simulink library "Library_SII_2018"  (R2018b)
settings: Solver=ode45  StartTime=0.0  StopTime=10.0  RelTol=1e-3  EnableMultiTasking=on
undefined symbols (not defined in the file or in its folder): coder, gcbh, r, simscape
libraries: fl_lib x157, nesl_utility x81, Library_SII2 x44, simulink x17, powerlib x12, mblibv1 x11, Simscape_SII_lib x11, elec_lib x10, Pneumatic_lib x4, $bdroot x2, peRmsMeasurement x1, powerlib_extras x1
(part 3 of 6)

== system Library_SII_2018/Electromécanique/Commande moteur Position ==
  cons pos : Inport
  pos codeur : Inport  Port=2
  Abs : Abs
  Constant : Constant  Value=0
  Controlled Voltage Source : fl_lib/Electrical/Electrical Sources/Controlled Voltage Source
  PID Controller : simulink/Continuous/PID Controller  Controller=PID  Form=Parallel  TimeDomain=Continuous-time  SampleTime=-1  IntegratorMethod=Forward Euler  FilterMethod=Forward Euler  ControllerParametersSource=internal  P=P  I=I  D=D  UseFilter=on  N=100  TunerSelectOption=Transfer Function Based (PID Tuner App)  InitialConditionSource=internal  InitialConditionForIntegrator=0  InitialConditionForFilter=0  DifferentiatorICPrevScaledInput=0  ExternalReset=either  TrackingMode=off  Kt=1  LimitOutput=on  UpperSaturationLimit=Umax  LowerSaturationLimit=-Umax  LinearizeAsGain=on  AntiWindupMode=none  Kb=1  POutMin=[]  POutMax=[]  IOutMin=[]  IOutMax=[]  DOutMin=[]  DOutMax=[]  NOutMin=[]  NOutMax=[]  SumOutMin=[]  SumOutMax=[]  SaturationOutMin=[]  SaturationOutMax=[]  PParamMin=[]  PParamMax=[]  IParamMin=[]  IParamMax=[]  DParamMin=[]  DParamMax=[]  NParamMin=[]  NParamMax=[]  KbParamMin=[]  KbParamMax=[]  KtParamMin=[]  KtParamMax=[]  KbOutMin=[]  KbOutMax=[]  KtOutMin=[]  KtOutMax=[]  IntegratorOutMin=[]  IntegratorOutMax=[]  FilterOutMin=[]  FilterOutMax=[]  SumI1OutMin=[]  SumI1OutMax=[]  SumI2OutMin=[]  SumI2OutMax=[]  SumI3OutMin=[]  SumI3OutMax=[]  SumI4OutMin=[]  SumI4OutMax=[]  SumDOutMin=[]  SumDOutMax=[]  DifferentiatorOutMin=[]  DifferentiatorOutMax=[]  FilterDiffOutCoefMin=[]  FilterDiffOutCoefMax=[]  ReciprocalOutMin=[]  ReciprocalOutMax=[]  SumDenOutMin=[]  SumDenOutMax=[]  SumNumOutMin=[]  SumNumOutMax=[]  DivideOutMin=[]  DivideOutMax=[]  IntegratorContinuousStateAttributes=''  IntegratorStateMustResolveToSignalObject=off  IntegratorRTWStateStorageClass=Auto  FilterContinuousStateAttributes=''  FilterStateMustResolveToSignalObject=off  FilterRTWStateStorageClass=Auto  ParallelPVariant=InternalParameters  IdealPVariant=Disabled  IVariant=InternalParameters  DVariant=InternalParameters  IntegratorVariant=Continuous  SatVariant=Enabled  AWVariant=Passthrough  PCopyVariant=Disabled  TRVariant=Disabled  FdbkBlocksVariant=Forward  IdealPFdbkVariant=Disabled  SatFdbkVariant=Disabled  DerivativeFilterVariant=ContFilter  NVariant=InternalParameters  NCopyVariant=Disabled  FilterICVariant=InternalICsFilter  IntegratorICVariant=InternalICs  ExternalResetVariant=ExternalReset  TRSumVariant=Passthrough  SumFdbkVariant=Disabled  SumVariant=Sum_PID
  Relay : Relay  OnSwitchValue=e  OffSwitchValue=e/2
  Simulink-PS Converter1 : nesl_utility/Simulink-PS Converter  PhysicalDomain=network_engine_domain  SubClassName=ps_input  LeftPortType=input  RightPortType=output  PseudoPeriodic=off  Frequencies=[]  NoiseDistribution=none  NoiseParameters=[]  Unit=1  AffineConversion=off  FilteringAndDerivatives=zero  SimscapeFilterOrder=1  InputFilterTimeConstant=0.001  UdotUserProvided=1
  Sum : Sum  Inputs=|+-
  Switch : Switch  Criteria=u2 > Threshold
  +mot : PMIOPort  Side=Right
  GND : PMIOPort  Port=2  Side=Right
  wires:
  pos codeur/1 -> Sum/2
  Switch/1 -> Simulink-PS Converter1/1, PID Controller/2
  Sum/1 -> Abs/1, PID Controller/1
  cons pos/1 -> Sum/1
  Constant/1 -> Switch/3
  Abs/1 -> Relay/1
  PID Controller/1 -> Switch/1
  Relay/1 -> Switch/2
  connections:
  GND/RConn1 -- Controlled Voltage Source/RConn2
  +mot/RConn1 -- Controlled Voltage Source/LConn1
  Simulink-PS Converter1/RConn1 -- Controlled Voltage Source/RConn1

== system Library_SII_2018/Electromécanique/Décodeur pour codeur incrémental ==
  A : Inport
  B : Inport  Port=2
  Clock1 : Clock
  Décodeur position - vitesse accélération - fréquence : Stateflow chart  TreatAsAtomicUnit=on
  MATLAB Function : MATLAB Function  TreatAsAtomicUnit=on
  Résolution : Constant  Value=r/2
  Terminator : Terminator
  Terminator1 : Terminator
  Terminator2 : Terminator
  inversion : Constant  Value=inv
  pos codeur : Outport
  wires:
  A/1 -> Décodeur position - vitesse accélération - fréquence/1(A), Décodeur position - vitesse accélération - fréquence/Trigger
  Clock1/1 -> Décodeur position - vitesse accélération - fréquence/4(t)
  B/1 -> Décodeur position - vitesse accélération - fréquence/2(B)
  Résolution/1 -> MATLAB Function/1(u)
  Décodeur position - vitesse accélération - fréquence/1(p) -> pos codeur/1
  Décodeur position - vitesse accélération - fréquence/2(v) -> Terminator/1
  Décodeur position - vitesse accélération - fréquence/4(f) -> Terminator2/1
  Décodeur position - vitesse accélération - fréquence/3(a) -> Terminator1/1
  MATLAB Function/1(y) -> Décodeur position - vitesse accélération - fréquence/3(k)
  inversion/1 -> MATLAB Function/2(inv)

== system Library_SII_2018/Electromécanique/Moteur CC (SPS-SM) ==
  Actionneur en vitesse : Subsystem
  Axe (inertie nulle) : mblibv1/Bodies/Body  LConnTagsString=CG  RConnTagsString=CS2  UpdateFromCAD=off  DialogClass=MechanicalBodyBlock  Mass=0.0001  MassUnits=kg  InertiaUnits=kg*m^2  Inertia=[1e-9 0 0 ; 0 1e-8 0 ; 0 0 1e-8]  Shape=Cylinder  ShapeDims=[1 1]  ShapeUnits=m  ShapeUse=false  Density=1  DensityUnits=kg/m^3  DensityUse=false  GraphicsMode=EQELLIPSE  BodyColorSelMode=COLORPALETTE  BodyColor=[0 1 0]  AttachedToCS=CG  CG=Left$CG$[0 0 0]$Adjoining$Adjoining$m$[0 0 0]$Euler X-Y-Z$deg$World$true$none  WorkingFrames=Right$CS2$[0 0 0]$CG$CG$mm$[0 0 0]$Euler X-Y-Z$deg$World$true$none  CGPos=[0 0 0]  CGRot=[0 0 0]  CS0Pos=[]  CS0Rot=[]  CS1Pos=[]  CS1Rot=[]  CS2Pos=[0 0 0]  CS2Rot=[0 0 0]  CS3Pos=[]  CS3Rot=[]  CS4Pos=[]  CS4Rot=[]  CS5Pos=[]  CS5Rot=[]  CS6Pos=[]  CS6Rot=[]  CS7Pos=[]  CS7Rot=[]  CS8Pos=[]  CS8Rot=[]  CS9Pos=[]  CS9Rot=[]  CS10Pos=[]  CS10Rot=[]  CS11Pos=[]  CS11Rot=[]  CS12Pos=[]  CS12Rot=[]  CS13Pos=[]  CS13Rot=[]  CS14Pos=[]  CS14Rot=[]  CS15Pos=[]  CS15Rot=[]  CS16Pos=[]  CS16Rot=[]  CS17Pos=[]  CS17Rot=[]  CS18Pos=[]  CS18Rot=[]  CS19Pos=[]  CS19Rot=[]  CS20Pos=[]  CS20Rot=[]
      settings: SourceProductName=Simscape Multibody  SourceProductBaseCode=MS
  Bus Selector : BusSelector  OutputSignals=Electrical torque Te (n m),Speed wm (rad/s)
  Capteur de couple : mblibv1/Sensors &  Actuators/Joint Sensor  UpdateFromCAD=off  PhysicalDomain=Mechanical  PortType=blob  Muxed=on  Pose=off  Angle=off  AngleUnits=deg  ArcVelocity=off  ArcVelocityUnits=deg/s  ArcAcceleration=off  ArcAccelerationUnits=deg/s^2  CoordPosition=on  CoordPositionUnits=m  Velocity=off  VelocityUnits=m/s  Acceleration=off  AccelerationUnits=m/s^2  Quaternion=on  QuaternionDT=off  QuaternionDDT=off  QuaternionUnits=off  OutputVector=[1]  ActiveIO=off  Width=3  DialogClass=MechanicalSensorBlock  Primitive=W  Force=off  ForceUnits=N  Torque=on  TorqueUnits=N*m  ReferenceFrame=Absolute (World)  ReactionSensedSide=Base  ReactionReferenceFrame=Absolute (World)  ReactionForce=off  ReactionForceUnits=N  ReactionMoment=on  ReactionMomentUnits=N*m
      settings: SourceProductName=Simscape Multibody  SourceProductBaseCode=MS
  Couple résistant : Scope
  Couple moteur : Scope
  DC Machine : powerlib/Machines/DC Machine  PresetModel=No  MechanicalLoad=Torque TL  FieldType=Permanent magnet  ShowDetailedParameters=on  MeasurementBus=off  RLa=[R L]  RLf=[281.3 156]  Laf=0.9483  MachineConstant=Back-emf constant (V/rpm)  Ke=K  Kt=1.8  J=J  Bm=kv  Tf=kc  w0=0  Ifinit=1  TsPowergui=0  TsBlock=-1
      settings: AttributesFormatString=\n  SourceProductName=Simscape Electrical
  Demux : Demux  Outputs=3
  Encastrement : mblibv1/Joints/Weld  LConnTagsString=__newl0|SA1  RConnTagsString=__newr0  UpdateFromCAD=off  NumSAPorts=1  CutJoint=off  MarkAsCut=off  Primitives=weld  PrimitiveProps=W$World$[0 0 0]$weld  DialogClass=JointBlock  WAxis=[0 0 0]
      settings: SourceProductName=Simscape Multibody  SourceProductBaseCode=MS
  Gain : Gain  Gain=-1
  Revolute : mblibv1/Joints/Revolute  LConnTagsString=__newl0|SA1  RConnTagsString=__newr0  UpdateFromCAD=off  NumSAPorts=1  CutJoint=off  MarkAsCut=off  Primitives=prismatic  PrimitiveProps=R1$World$[1 0 0]$revolute  DialogClass=JointBlock  R1Axis=[1 0 0]
      settings: SourceProductName=Simscape Multibody  SourceProductBaseCode=MS
  T : Terminator
  T1 : Terminator
  Stator : PMIOPort  Side=Left
  Rotor : PMIOPort  Port=2  Side=Right
  A+ : PMIOPort  Port=3  Side=Left
  A- : PMIOPort  Port=4  Side=Right
  wires:
  Bus Selector/2 -> Actionneur en vitesse/1(signal)  "<Speed wm (rad/s)>"
  Demux/3 -> T1/1
  Demux/2 -> T/1  "Couple"
  Demux/1 -> Gain/1
  Gain/1 -> Couple résistant/1, DC Machine/1
  Bus Selector/1 -> Couple moteur/1  "<Electrical torque Te (n m)>"
  Capteur de couple/1 -> Demux/1
  DC Machine/1 -> Bus Selector/1
  connections:
  A-/RConn1 -- DC Machine/RConn1
  A+/RConn1 -- DC Machine/LConn1
  Stator/RConn1 -- Revolute/LConn1
  Actionneur en vitesse/RConn1 -- Revolute/LConn2
  Encastrement/RConn1 -- Rotor/RConn1
  Capteur de couple/LConn1 -- Encastrement/LConn2
  Axe (inertie nulle)/RConn1 -- Encastrement/LConn1
  Revolute/RConn1 -- Axe (inertie nulle)/LConn1

== system Library_SII_2018/Electromécanique/Moteur CC (SPS-SS) ==
  Bus Selector : BusSelector  OutputSignals=Electrical torque Te (n m),Speed wm (rad/s)
  Capteur de couple : fl_lib/Mechanical/Mechanical Sensors/Ideal Torque Sensor
  Couple résistant : Scope
  Couple moteur : Scope
  DC Machine : powerlib/Machines/DC Machine  PresetModel=No  MechanicalLoad=Torque TL  FieldType=Permanent magnet  ShowDetailedParameters=on  MeasurementBus=off  RLa=[R L]  RLf=[281.3 156]  Laf=0.9483  MachineConstant=Back-emf constant (V/rpm)  Ke=K  Kt=1.8  J=J  Bm=kv  Tf=kc  w0=0  Ifinit=1  TsPowergui=0  TsBlock=-1
      settings: AttributesFormatString=\n  SourceProductName=Simscape Electrical
  Frottement visqueux : fl_lib/Mechanical/Rotational Elements/Rotational Damper  D=kv N*m/(rad/s)  w_specify=off  w_priority=High  w=0 rad/s  w_nominal_specify=off  w_nominal_unit=rad/s  w_nominal_value=1  t_specify=off  t_priority=High  t=0 N*m  t_nominal_specify=off  t_nominal_unit=N*m  t_nominal_value=1
  Gain : Gain  Gain=-1
  Inertie arbre : fl_lib/Mechanical/Rotational Elements/Inertia  inertia=J kg*m^2  w_specify=on  w_priority=High  w=0 rad/s  w_nominal_specify=off  w_nominal_unit=rad/s  w_nominal_value=1  t_specify=off  t_priority=High  t=0 N*m  t_nominal_specify=off  t_nominal_unit=N*m  t_nominal_value=1
  Mechanical Rotational Reference : fl_lib/Mechanical/Rotational Elements/Mechanical Rotational Reference
  PS-Simulink Converter : nesl_utility/PS-Simulink Converter  PhysicalDomain=network_engine_domain  SubClassName=ps_output  LeftPortType=input  RightPortType=output  PseudoPeriodic=off  Frequencies=[]  Unit=1  AffineConversion=off
  Ref : fl_lib/Mechanical/Rotational Elements/Mechanical Rotational Reference
  Ref Stator : fl_lib/Mechanical/Rotational Elements/Mechanical Rotational Reference
  Simulink-PS Converter : nesl_utility/Simulink-PS Converter  PhysicalDomain=network_engine_domain  SubClassName=ps_input  LeftPortType=input  RightPortType=output  PseudoPeriodic=off  Frequencies=[]  NoiseDistribution=none  NoiseParameters=[]  Unit=1  AffineConversion=off  FilteringAndDerivatives=zero  SimscapeFilterOrder=1  InputFilterTimeConstant=.001  UdotUserProvided=0
  Solver Configuration : nesl_utility/Solver Configuration  PhysicalDomain=network_engine_domain  SubClassName=solver  LeftPortType=input  RightPortType=generic  Tones=[]  Harmonics=[]  SimulateNoise=off  Profile=off  UseLocalSampling=off  EnableSwitchedLinearOptims=on  FrequencyDomain=off  UseCCode=off  RelTol=0.001  AbsTol=1e-06  MinStep=1e-09  ToWorkspace=off  RevertToSquareIcSolve=off  NumHomotopyIterations=100  PhasorMode=off  PhasorModeNumHarmonics=1  DoDC=off  ResidualTolerance=1e-9  UseLocalSolver=off  LocalSolverChoice=NE_BACKWARD_EULER_ADVANCER  LocalSolverSampleTime=.001  DoFixedCost=off  MaxNonlinIter=3  MaxModeIter=2  LinearAlgebra=Sparse  EquationFormulation=NE_TIME_EF  DelaysMemoryBudget=1024  AutomaticFiltering=on  FilteringTimeConstant=0.001  PartitionStorageMethod=AS_NEEDED  PartitionMemoryBudget=1024
  Source de vitesse : fl_lib/Mechanical/Mechanical Sources/Ideal Angular Velocity Source
  Stator : PMIOPort  Side=Left
  Rotor : PMIOPort  Port=2  Side=Right
  A+ : PMIOPort  Port=3  Side=Left
  A- : PMIOPort  Port=4  Side=Right
  wires:
  Bus Selector/2 -> Simulink-PS Converter/1  "<Speed wm (rad/s)>"
  PS-Simulink Converter/1 -> Gain/1
  Gain/1 -> Couple résistant/1, DC Machine/1
  Bus Selector/1 -> Couple moteur/1  "<Electrical torque Te (n m)>"
  DC Machine/1 -> Bus Selector/1
  connections:
  Capteur de couple/RConn1 -- Source de vitesse/LConn1 -- Frottement visqueux/RConn1 -- Inertie arbre/LConn1
  Mechanical Rotational Reference/LConn1 -- Source de vitesse/RConn2
  Ref/LConn1 -- Frottement visqueux/LConn1
  Capteur de couple/LConn1 -- Solver Configuration/RConn1 -- Rotor/RConn1
  Capteur de couple/RConn2 -- PS-Simulink Converter/LConn1
  Ref Stator/LConn1 -- Stator/RConn1
  Source de vitesse/RConn1 -- Simulink-PS Converter/RConn1
  A-/RConn1 -- DC Machine/RConn1
  A+/RConn1 -- DC Machine/LConn1

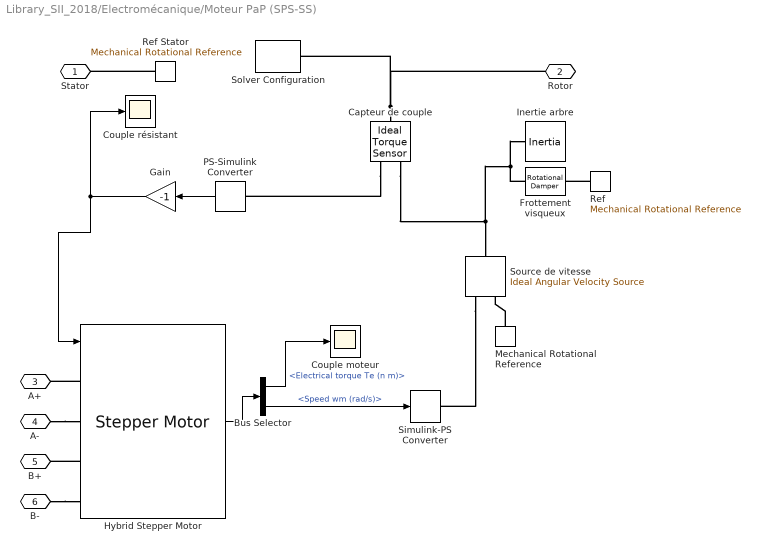
== system Library_SII_2018/Electromécanique/Moteur PaP (SPS-SS) ==
  Bus Selector : BusSelector  OutputSignals=Electrical torque Te (n m),Speed wm (rad/s)
  Capteur de couple : fl_lib/Mechanical/Mechanical Sensors/Ideal Torque Sensor
  Couple résistant : Scope
  Couple moteur : Scope
  Frottement visqueux : fl_lib/Mechanical/Rotational Elements/Rotational Damper  D=kv N*m/(rad/s)  w_specify=off  w_priority=High  w=0 rad/s  w_nominal_specify=off  w_nominal_unit=rad/s  w_nominal_value=1  t_specify=off  t_priority=High  t=0 N*m  t_nominal_specify=off  t_nominal_unit=N*m  t_nominal_value=1
  Gain : Gain  Gain=-1
  Hybrid Stepper Motor : powerlib/Machines/Stepper Motor  MotorType=Permanent-magnet / Hybrid  NumberOfPhases_1=2  NumberOfPhases_2=3  PresetModel_1=<empty>  PresetModel_2=<empty>  L=1.4e-3  Lmax=10e-3  Lmin=2e-3  R=0.7  Step_angle=1.8  Psim=0.005  Tdm=0.002  J=1.2e-7  B=1e-7*1000  w0=0  pos0=0  TsPowergui=0  TsBlock=-1
      settings: SourceProductName=Simscape Electrical  SourceProductBaseCode=PS
  Inertie arbre : fl_lib/Mechanical/Rotational Elements/Inertia  inertia=J kg*m^2  w_specify=on  w_priority=High  w=0 rad/s  w_nominal_specify=off  w_nominal_unit=rad/s  w_nominal_value=1  t_specify=off  t_priority=High  t=0 N*m  t_nominal_specify=off  t_nominal_unit=N*m  t_nominal_value=1
  Mechanical Rotational Reference : fl_lib/Mechanical/Rotational Elements/Mechanical Rotational Reference
  PS-Simulink Converter : nesl_utility/PS-Simulink Converter  PhysicalDomain=network_engine_domain  SubClassName=ps_output  LeftPortType=input  RightPortType=output  PseudoPeriodic=off  Frequencies=[]  Unit=1  AffineConversion=off
  Ref : fl_lib/Mechanical/Rotational Elements/Mechanical Rotational Reference
  Ref Stator : fl_lib/Mechanical/Rotational Elements/Mechanical Rotational Reference
  Simulink-PS Converter : nesl_utility/Simulink-PS Converter  PhysicalDomain=network_engine_domain  SubClassName=ps_input  LeftPortType=input  RightPortType=output  PseudoPeriodic=off  Frequencies=[]  NoiseDistribution=none  NoiseParameters=[]  Unit=1  AffineConversion=off  FilteringAndDerivatives=zero  SimscapeFilterOrder=1  InputFilterTimeConstant=.001  UdotUserProvided=0
  Solver Configuration : nesl_utility/Solver Configuration  PhysicalDomain=network_engine_domain  SubClassName=solver  LeftPortType=input  RightPortType=generic  Tones=[]  Harmonics=[]  SimulateNoise=off  Profile=off  UseLocalSampling=off  EnableSwitchedLinearOptims=on  FrequencyDomain=off  UseCCode=off  RelTol=0.001  AbsTol=1e-06  MinStep=1e-09  ToWorkspace=off  RevertToSquareIcSolve=off  NumHomotopyIterations=100  PhasorMode=off  PhasorModeNumHarmonics=1  DoDC=off  ResidualTolerance=1e-9  UseLocalSolver=off  LocalSolverChoice=NE_BACKWARD_EULER_ADVANCER  LocalSolverSampleTime=.001  DoFixedCost=off  MaxNonlinIter=3  MaxModeIter=2  LinearAlgebra=Sparse  EquationFormulation=NE_TIME_EF  DelaysMemoryBudget=1024  AutomaticFiltering=on  FilteringTimeConstant=0.001  PartitionStorageMethod=AS_NEEDED  PartitionMemoryBudget=1024
  Source de vitesse : fl_lib/Mechanical/Mechanical Sources/Ideal Angular Velocity Source
  Stator : PMIOPort  Side=Left
  Rotor : PMIOPort  Port=2  Side=Right
  A+ : PMIOPort  Port=3  Side=Left
  A- : PMIOPort  Port=4  Side=Right
  B+ : PMIOPort  Port=5  Side=Left
  B- : PMIOPort  Port=6  Side=Right
  wires:
  Bus Selector/2 -> Simulink-PS Converter/1  "<Speed wm (rad/s)>"
  PS-Simulink Converter/1 -> Gain/1
  Gain/1 -> Hybrid Stepper Motor/1, Couple résistant/1
  Bus Selector/1 -> Couple moteur/1  "<Electrical torque Te (n m)>"
  Hybrid Stepper Motor/1 -> Bus Selector/1
  connections:
  Capteur de couple/RConn1 -- Source de vitesse/LConn1 -- Frottement visqueux/RConn1 -- Inertie arbre/LConn1
  Mechanical Rotational Reference/LConn1 -- Source de vitesse/RConn2
  Ref/LConn1 -- Frottement visqueux/LConn1
  Capteur de couple/LConn1 -- Solver Configuration/RConn1 -- Rotor/RConn1
  Capteur de couple/RConn2 -- PS-Simulink Converter/LConn1
  Ref Stator/LConn1 -- Stator/RConn1
  Source de vitesse/RConn1 -- Simulink-PS Converter/RConn1
  A-/RConn1 -- Hybrid Stepper Motor/LConn2
  Hybrid Stepper Motor/LConn1 -- A+/RConn1
  Hybrid Stepper Motor/LConn3 -- B+/RConn1
  B-/RConn1 -- Hybrid Stepper Motor/LConn4

== system Library_SII_2018/Electromécanique/Pont en H ==
  mode : Inport
  Commande du pont en H : MATLAB Function  TreatAsAtomicUnit=on
  Simulink-PS Converter{1,3..5} (4 alike) : nesl_utility/Simulink-PS Converter  PhysicalDomain=network_engine_domain  SubClassName=ps_input  LeftPortType=input  RightPortType=output  PseudoPeriodic=off  Frequencies=[]  NoiseDistribution=none  NoiseParameters=[]  Unit=V  AffineConversion=off  FilteringAndDerivatives=zero  SimscapeFilterOrder=1  InputFilterTimeConstant=0.1  UdotUserProvided=1
  a : fl_lib/Electrical/Electrical Elements/Switch  R_closed=0.01 Ohm  G_open=1e-8 1/Ohm  Threshold=0.5  i_specify=off  i_priority=High  i=0 A  i_nominal_specify=off  i_nominal_unit=A  i_nominal_value=1  v_specify=off  v_priority=High  v=0 V  v_nominal_specify=off  v_nominal_unit=V  v_nominal_value=1
      settings: SourceProductName=Simscape
  b : fl_lib/Electrical/Electrical Elements/Switch  R_closed=0.01 Ohm  G_open=1e-8 1/Ohm  Threshold=0.5  i_specify=off  i_priority=High  i=0 A  i_nominal_specify=off  i_nominal_unit=A  i_nominal_value=1  v_specify=off  v_priority=High  v=0 V  v_nominal_specify=off  v_nominal_unit=V  v_nominal_value=1
      settings: SourceProductName=Simscape
  c : fl_lib/Electrical/Electrical Elements/Switch  R_closed=0.01 Ohm  G_open=1e-8 1/Ohm  Threshold=0.5  i_specify=off  i_priority=High  i=0 A  i_nominal_specify=off  i_nominal_unit=A  i_nominal_value=1  v_specify=off  v_priority=High  v=0 V  v_nominal_specify=off  v_nominal_unit=V  v_nominal_value=1
      settings: SourceProductName=Simscape
  d : fl_lib/Electrical/Electrical Elements/Switch  R_closed=0.01 Ohm  G_open=1e-8 1/Ohm  Threshold=0.5  i_specify=off  i_priority=High  i=0 A  i_nominal_specify=off  i_nominal_unit=A  i_nominal_value=1  v_specify=off  v_priority=High  v=0 V  v_nominal_specify=off  v_nominal_unit=V  v_nominal_value=1
      settings: SourceProductName=Simscape
  Vcc : PMIOPort  Side=Left
  +Mot : PMIOPort  Port=2  Side=Right
  -Mot : PMIOPort  Port=3  Side=Right
  Ref : PMIOPort  Port=4  Side=Left
  wires:
  Commande du pont en H/1(a) -> Simulink-PS Converter1/1
  Commande du pont en H/3(c) -> Simulink-PS Converter5/1
  Commande du pont en H/4(d) -> Simulink-PS Converter4/1
  mode/1 -> Commande du pont en H/1(mode)
  Commande du pont en H/2(b) -> Simulink-PS Converter3/1
  connections:
  a/LConn1 -- +Mot/RConn1 -- c/RConn2
  Simulink-PS Converter1/RConn1 -- a/RConn1
  Simulink-PS Converter5/RConn1 -- c/RConn1
  b/RConn2 -- Vcc/RConn1 -- a/RConn2
  Simulink-PS Converter3/RConn1 -- b/RConn1
  d/LConn1 -- Ref/RConn1 -- c/LConn1
  Simulink-PS Converter4/RConn1 -- d/RConn1
  b/LConn1 -- -Mot/RConn1 -- d/RConn2

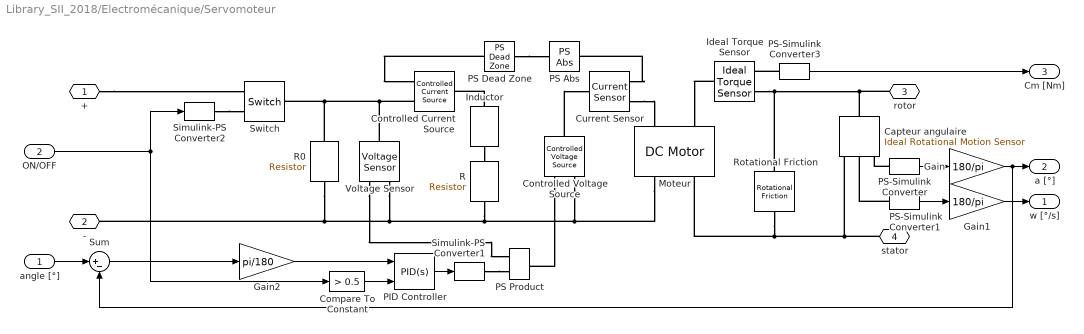
== system Library_SII_2018/Electromécanique/Servomoteur ==
  angle [°] : Inport
  ON/OFF : Inport  Port=2
  Capteur angulaire : fl_lib/Mechanical/Mechanical Sensors/Ideal Rotational Motion Sensor  offset=0 rad
  Compare To Constant : simulink/Logic and Bit Operations/Compare To Constant  relop=>  const=0.5  OutDataTypeStr=boolean
  Controlled Current Source : fl_lib/Electrical/Electrical Sources/Controlled Current Source
  Controlled Voltage Source : fl_lib/Electrical/Electrical Sources/Controlled Voltage Source
  Current Sensor : fl_lib/Electrical/Electrical Sensors/Current Sensor
  Gain : Gain  Gain=180/pi
  Gain1 : Gain  Gain=180/pi
  Gain2 : Gain  Gain=pi/180
  Ideal Torque Sensor : fl_lib/Mechanical/Mechanical Sensors/Ideal Torque Sensor
  Inductor : fl_lib/Electrical/Electrical Elements/Inductor  l=L H  r=0 Ohm  g=1e-9 1/Ohm  i_specify=off  i_priority=High  i=0 A  i_nominal_specify=off  i_nominal_unit=A  i_nominal_value=1  v_specify=off  v_priority=High  v=0 V  v_nominal_specify=off  v_nominal_unit=V  v_nominal_value=1  i_L_specify=off  i_L_priority=High  i_L=0 A  i_L_nominal_specify=off  i_L_nominal_unit=A  i_L_nominal_value=1
  Moteur : elec_lib/Actuators & Drivers/Rotational Actuators/DC Motor  parameterization=1  Ra=R Ohm  La=L H  emf_or_torque=1  Kv=K V/(rad/s)  Ki=6.876e-4 N*m/A  T_stall=2.4e-4 N*m  w_max=1.91e+4 rpm  w_rated=1.5e+4 rpm  P_rated=0.08 W  V_rated=1.5 V  J=0.001 g*cm^2  lam_param=1  lam=kv N*m/(rad/s)  i_noload=0 A  V_i_noload=1.5 V  speed0=0 rpm  alpha=0.00393 1/K  Tmeas=25 C  thermal_mass=100 J/K  initial_temperature=25 C
  PID Controller : simulink/Continuous/PID Controller  Controller=PID  Form=Ideal  TimeDomain=Continuous-time  SampleTime=-1  IntegratorMethod=Forward Euler  FilterMethod=Forward Euler  ControllerParametersSource=internal  P=P  I=I  D=D  UseFilter=on  N=100  TunerSelectOption=Transfer Function Based (PID Tuner App)  InitialConditionSource=internal  InitialConditionForIntegrator=0  InitialConditionForFilter=0  DifferentiatorICPrevScaledInput=0  ExternalReset=rising  TrackingMode=off  Kt=1  LimitOutput=on  UpperSaturationLimit=1  LowerSaturationLimit=-1  LinearizeAsGain=on  AntiWindupMode=none  Kb=1  POutMin=[]  POutMax=[]  IOutMin=[]  IOutMax=[]  DOutMin=[]  DOutMax=[]  NOutMin=[]  NOutMax=[]  SumOutMin=[]  SumOutMax=[]  SaturationOutMin=[]  SaturationOutMax=[]  PParamMin=[]  PParamMax=[]  IParamMin=[]  IParamMax=[]  DParamMin=[]  DParamMax=[]  NParamMin=[]  NParamMax=[]  KbParamMin=[]  KbParamMax=[]  KtParamMin=[]  KtParamMax=[]  KbOutMin=[]  KbOutMax=[]  KtOutMin=[]  KtOutMax=[]  IntegratorOutMin=[]  IntegratorOutMax=[]  FilterOutMin=[]  FilterOutMax=[]  SumI1OutMin=[]  SumI1OutMax=[]  SumI2OutMin=[]  SumI2OutMax=[]  SumI3OutMin=[]  SumI3OutMax=[]  SumI4OutMin=[]  SumI4OutMax=[]  SumDOutMin=[]  SumDOutMax=[]  DifferentiatorOutMin=[]  DifferentiatorOutMax=[]  FilterDiffOutCoefMin=[]  FilterDiffOutCoefMax=[]  ReciprocalOutMin=[]  ReciprocalOutMax=[]  SumDenOutMin=[]  SumDenOutMax=[]  SumNumOutMin=[]  SumNumOutMax=[]  DivideOutMin=[]  DivideOutMax=[]  IntegratorContinuousStateAttributes=''  IntegratorStateMustResolveToSignalObject=off  IntegratorRTWStateStorageClass=Auto  FilterContinuousStateAttributes=''  FilterStateMustResolveToSignalObject=off  FilterRTWStateStorageClass=Auto  ParallelPVariant=Passthrough  IdealPVariant=InternalParameters  IVariant=InternalParameters  DVariant=InternalParameters  IntegratorVariant=Continuous  SatVariant=Enabled  AWVariant=Passthrough  PCopyVariant=Disabled  TRVariant=Disabled  FdbkBlocksVariant=Forward  IdealPFdbkVariant=Disabled  SatFdbkVariant=Disabled  DerivativeFilterVariant=ContFilter  NVariant=InternalParameters  NCopyVariant=Disabled  FilterICVariant=InternalICsFilter  IntegratorICVariant=InternalICs  ExternalResetVariant=ExternalReset  TRSumVariant=Passthrough  SumFdbkVariant=Disabled  SumVariant=Sum_PID
  PS Abs : fl_lib/Physical Signals/Nonlinear Operators/PS Abs
      settings: SourceProductName=Simscape  SourceProductBaseCode=SS
  PS Dead Zone : fl_lib/Physical Signals/Nonlinear Operators/PS Dead Zone  upper_limit=0.01  lower_limit=- 0.01
      settings: SourceProductName=Simscape  SourceProductBaseCode=SS
  PS Product : fl_lib/Physical Signals/Functions/PS Product
      settings: SourceProductName=Simscape
  PS-Simulink Converter : nesl_utility/PS-Simulink Converter  PhysicalDomain=network_engine_domain  SubClassName=ps_output  LeftPortType=input  RightPortType=output  PseudoPeriodic=off  Frequencies=[]  Unit=1  AffineConversion=off
  PS-Simulink Converter1 : nesl_utility/PS-Simulink Converter  PhysicalDomain=network_engine_domain  SubClassName=ps_output  LeftPortType=input  RightPortType=output  PseudoPeriodic=off  Frequencies=[]  Unit=1  AffineConversion=off
  PS-Simulink Converter3 : nesl_utility/PS-Simulink Converter  PhysicalDomain=network_engine_domain  SubClassName=ps_output  LeftPortType=input  RightPortType=output  PseudoPeriodic=off  Frequencies=[]  Unit=1  AffineConversion=off
  R : fl_lib/Electrical/Electrical Elements/Resistor  R=R Ohm  i_specify=off  i_priority=High  i=0 A  i_nominal_specify=off  i_nominal_unit=A  i_nominal_value=1  v_specify=off  v_priority=High  v=0 V  v_nominal_specify=off  v_nominal_unit=V  v_nominal_value=1
  R0 : fl_lib/Electrical/Electrical Elements/Resistor  R=R0 Ohm  i_specify=off  i_priority=High  i=0 A  i_nominal_specify=off  i_nominal_unit=A  i_nominal_value=1  v_specify=off  v_priority=High  v=0 V  v_nominal_specify=off  v_nominal_unit=V  v_nominal_value=1
  Rotational Friction : fl_lib/Mechanical/Rotational Elements/Rotational Friction  brkwy_trq=Cf*1.1 N*m  brkwy_vel=0.060623 rad/s  Col_trq=Cf N*m  visc_coef=0.0001 N*m/(rad/s)  w_specify=off  w_priority=High  w=0 rad/s  w_nominal_specify=off  w_nominal_unit=rad/s  w_nominal_value=1  t_specify=off  t_priority=High  t=0 N*m  t_nominal_specify=off  t_nominal_unit=N*m  t_nominal_value=1
      settings: SourceProductName=Simscape
  Simulink-PS Converter1 : nesl_utility/Simulink-PS Converter  PhysicalDomain=network_engine_domain  SubClassName=ps_input  LeftPortType=input  RightPortType=output  PseudoPeriodic=off  Frequencies=[]  NoiseDistribution=none  NoiseParameters=[]  Unit=V  AffineConversion=off  FilteringAndDerivatives=zero  SimscapeFilterOrder=1  InputFilterTimeConstant=0.1  UdotUserProvided=1
  Simulink-PS Converter2 : nesl_utility/Simulink-PS Converter  PhysicalDomain=network_engine_domain  SubClassName=ps_input  LeftPortType=input  RightPortType=output  PseudoPeriodic=off  Frequencies=[]  NoiseDistribution=none  NoiseParameters=[]  Unit=V  AffineConversion=off  FilteringAndDerivatives=zero  SimscapeFilterOrder=1  InputFilterTimeConstant=0.1  UdotUserProvided=1
  Sum : Sum  Inputs=|+-
  Switch : fl_lib/Electrical/Electrical Elements/Switch  R_closed=0.01 Ohm  G_open=1e-8 1/Ohm  Threshold=0.5  i_specify=off  i_priority=High  i=0 A  i_nominal_specify=off  i_nominal_unit=A  i_nominal_value=1  v_specify=off  v_priority=High  v=0 V  v_nominal_specify=off  v_nominal_unit=V  v_nominal_value=1
      settings: SourceProductName=Simscape
  Voltage Sensor : fl_lib/Electrical/Electrical Sensors/Voltage Sensor
  + : PMIOPort  Side=Left
  - : PMIOPort  Port=2  Side=Left
  rotor : PMIOPort  Port=3  Side=Right
  stator : PMIOPort  Port=4  Side=Right
  w [°/s] : Outport
  a [°] : Outport  Port=2
  Cm [Nm] : Outport  Port=3
  wires:
  PID Controller/1 -> Simulink-PS Converter1/1
  Gain1/1 -> w [°/s]/1
  PS-Simulink Converter/1 -> Gain/1
  PS-Simulink Converter1/1 -> Gain1/1
  Gain2/1 -> PID Controller/1
  angle [°]/1 -> Sum/1
  Gain/1 -> Sum/2, a [°]/1
  Sum/1 -> Gain2/1
  ON/OFF/1 -> Simulink-PS Converter2/1, Compare To Constant/1
  Compare To Constant/1 -> PID Controller/2
  PS-Simulink Converter3/1 -> Cm [Nm]/1
  connections:
  Inductor/RConn1 -- R/LConn1
  Inductor/LConn1 -- Controlled Current Source/LConn1
  Current Sensor/RConn1 -- PS Abs/LConn1
  Current Sensor/RConn2 -- Moteur/LConn1
  Controlled Current Source/RConn2 -- Voltage Sensor/LConn1 -- Switch/LConn1 -- R0/LConn1
  Controlled Voltage Source/LConn1 -- Current Sensor/LConn1
  Voltage Sensor/RConn2 -- R/RConn1 -- Controlled Voltage Source/RConn2 -- Moteur/RConn1 -- -/RConn1 -- R0/RConn1
  rotor/RConn1 -- Rotational Friction/LConn1 -- Ideal Torque Sensor/RConn1 -- Capteur angulaire/LConn1
  PS-Simulink Converter/LConn1 -- Capteur angulaire/RConn3
  PS-Simulink Converter1/LConn1 -- Capteur angulaire/RConn2
  Capteur angulaire/RConn1 -- Moteur/RConn2 -- Rotational Friction/RConn1 -- stator/RConn1
  PS Dead Zone/LConn1 -- PS Abs/RConn1
  Controlled Voltage Source/RConn1 -- PS Product/RConn1
  Simulink-PS Converter1/RConn1 -- PS Product/LConn2
  Voltage Sensor/RConn1 -- PS Product/LConn1
  +/RConn1 -- Switch/RConn2
  Simulink-PS Converter2/RConn1 -- Switch/RConn1
  PS Dead Zone/RConn1 -- Controlled Current Source/RConn1
  Ideal Torque Sensor/LConn1 -- Moteur/LConn2
  PS-Simulink Converter3/LConn1 -- Ideal Torque Sensor/RConn2

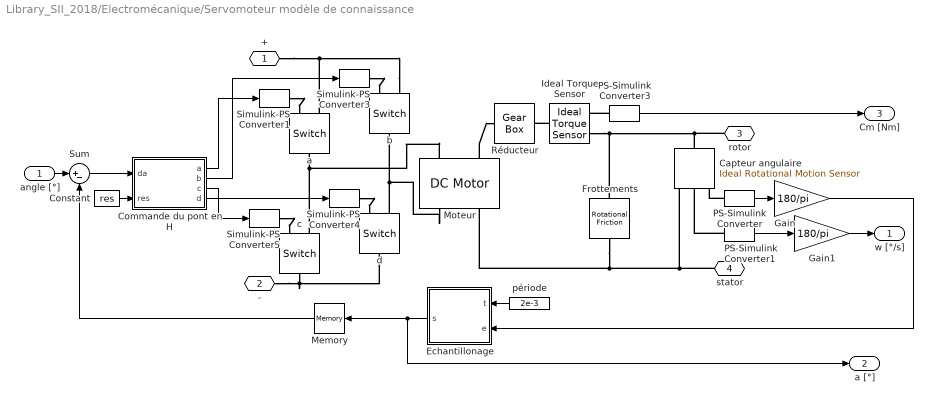
== system Library_SII_2018/Electromécanique/Servomoteur modèle de connaissance ==
  angle [°] : Inport
  Capteur angulaire : fl_lib/Mechanical/Mechanical Sensors/Ideal Rotational Motion Sensor  offset=0 rad
  Commande du pont en H : MATLAB Function  TreatAsAtomicUnit=on
      settings: MinAlgLoopOccurrences=on
  Constant : Constant  Value=res
  Echantillonage : Stateflow chart  TreatAsAtomicUnit=on
  Frottements : fl_lib/Mechanical/Rotational Elements/Rotational Friction  brkwy_trq=0.0194*1.1 N*m  brkwy_vel=0.060623 rad/s  Col_trq=0.0194 N*m  visc_coef=0.0001 N*m/(rad/s)  w_specify=off  w_priority=High  w=0 rad/s  w_nominal_specify=off  w_nominal_unit=rad/s  w_nominal_value=1  t_specify=off  t_priority=High  t=0 N*m  t_nominal_specify=off  t_nominal_unit=N*m  t_nominal_value=1
      settings: SourceProductName=Simscape
  Gain : Gain  Gain=180/pi
  Gain1 : Gain  Gain=180/pi
  Ideal Torque Sensor : fl_lib/Mechanical/Mechanical Sensors/Ideal Torque Sensor
  Memory : Memory  InheritSampleTime=on
  Moteur : elec_lib/Actuators & Drivers/Rotational Actuators/DC Motor  parameterization=2  Ra=1 Ohm  La=1e-5 H  emf_or_torque=1  Kv=1 V/(rad/s)  Ki=6.876e-4 N*m/A  T_stall=1.61e-3 N*m  w_max=12600 rpm  w_rated=1.5e+4 rpm  P_rated=0.08 W  V_rated=4.5 V  J=0.001 g*cm^2  lam_param=2  lam=0.000001 N*m/(rad/s)  i_noload=0.59 A  V_i_noload=4.5 V  speed0=0 rpm  alpha=0.00393 1/K  Tmeas=25 C  thermal_mass=100 J/K  initial_temperature=25 C
  PS-Simulink Converter : nesl_utility/PS-Simulink Converter  PhysicalDomain=network_engine_domain  SubClassName=ps_output  LeftPortType=input  RightPortType=output  PseudoPeriodic=off  Frequencies=[]  Unit=1  AffineConversion=off
  PS-Simulink Converter1 : nesl_utility/PS-Simulink Converter  PhysicalDomain=network_engine_domain  SubClassName=ps_output  LeftPortType=input  RightPortType=output  PseudoPeriodic=off  Frequencies=[]  Unit=1  AffineConversion=off
  PS-Simulink Converter3 : nesl_utility/PS-Simulink Converter  PhysicalDomain=network_engine_domain  SubClassName=ps_output  LeftPortType=input  RightPortType=output  PseudoPeriodic=off  Frequencies=[]  Unit=1  AffineConversion=off
  Réducteur : fl_lib/Mechanical/Mechanisms/Gear Box  ratio=278  t_in_specify=off  t_in_priority=High  t_in=0 N*m  t_in_nominal_specify=off  t_in_nominal_unit=N*m  t_in_nominal_value=1  t_out_specify=off  t_out_priority=High  t_out=0 N*m  t_out_nominal_specify=off  t_out_nominal_unit=N*m  t_out_nominal_value=1
  Simulink-PS Converter{1,3..5} (4 alike) : nesl_utility/Simulink-PS Converter  PhysicalDomain=network_engine_domain  SubClassName=ps_input  LeftPortType=input  RightPortType=output  PseudoPeriodic=off  Frequencies=[]  NoiseDistribution=none  NoiseParameters=[]  Unit=V  AffineConversion=off  FilteringAndDerivatives=zero  SimscapeFilterOrder=1  InputFilterTimeConstant=0.1  UdotUserProvided=1
  Sum : Sum  Inputs=|+-
  a : fl_lib/Electrical/Electrical Elements/Switch  R_closed=0.01 Ohm  G_open=1e-8 1/Ohm  Threshold=0.5  i_specify=off  i_priority=High  i=0 A  i_nominal_specify=off  i_nominal_unit=A  i_nominal_value=1  v_specify=off  v_priority=High  v=0 V  v_nominal_specify=off  v_nominal_unit=V  v_nominal_value=1
      settings: SourceProductName=Simscape
  b : fl_lib/Electrical/Electrical Elements/Switch  R_closed=0.01 Ohm  G_open=1e-8 1/Ohm  Threshold=0.5  i_specify=off  i_priority=High  i=0 A  i_nominal_specify=off  i_nominal_unit=A  i_nominal_value=1  v_specify=off  v_priority=High  v=0 V  v_nominal_specify=off  v_nominal_unit=V  v_nominal_value=1
      settings: SourceProductName=Simscape
  c : fl_lib/Electrical/Electrical Elements/Switch  R_closed=0.01 Ohm  G_open=1e-8 1/Ohm  Threshold=0.5  i_specify=off  i_priority=High  i=0 A  i_nominal_specify=off  i_nominal_unit=A  i_nominal_value=1  v_specify=off  v_priority=High  v=0 V  v_nominal_specify=off  v_nominal_unit=V  v_nominal_value=1
      settings: SourceProductName=Simscape
  d : fl_lib/Electrical/Electrical Elements/Switch  R_closed=0.01 Ohm  G_open=1e-8 1/Ohm  Threshold=0.5  i_specify=off  i_priority=High  i=0 A  i_nominal_specify=off  i_nominal_unit=A  i_nominal_value=1  v_specify=off  v_priority=High  v=0 V  v_nominal_specify=off  v_nominal_unit=V  v_nominal_value=1
      settings: SourceProductName=Simscape
  période : Constant  Value=2e-3
  + : PMIOPort  Side=Left
  - : PMIOPort  Port=2  Side=Left
  rotor : PMIOPort  Port=3  Side=Right
  stator : PMIOPort  Port=4  Side=Right
  w [°/s] : Outport
  a [°] : Outport  Port=2
  Cm [Nm] : Outport  Port=3
  wires:
  PS-Simulink Converter3/1 -> Cm [Nm]/1
  période/1 -> Echantillonage/1(t)
  Echantillonage/1(s) -> Memory/1, a [°]/1
  Constant/1 -> Commande du pont en H/2(res)
  Commande du pont en H/4(d) -> Simulink-PS Converter4/1
  Commande du pont en H/3(c) -> Simulink-PS Converter5/1
  Commande du pont en H/2(b) -> Simulink-PS Converter3/1
  Commande du pont en H/1(a) -> Simulink-PS Converter1/1
  Sum/1 -> Commande du pont en H/1(da)
  Gain1/1 -> w [°/s]/1
  PS-Simulink Converter/1 -> Gain/1
  PS-Simulink Converter1/1 -> Gain1/1
  angle [°]/1 -> Sum/1
  Gain/1 -> Echantillonage/2(e)
  Memory/1 -> Sum/2
  connections:
  Ideal Torque Sensor/LConn1 -- Réducteur/RConn1
  PS-Simulink Converter3/LConn1 -- Ideal Torque Sensor/RConn2
  Simulink-PS Converter5/RConn1 -- c/RConn1
  Simulink-PS Converter4/RConn1 -- d/RConn1
  Simulink-PS Converter3/RConn1 -- b/RConn1
  b/LConn1 -- d/RConn2 -- Moteur/RConn1
  a/LConn1 -- c/RConn2 -- Moteur/LConn1
  b/RConn2 -- +/RConn1 -- a/RConn2
  -/RConn1 -- d/LConn1 -- c/LConn1
  Simulink-PS Converter1/RConn1 -- a/RConn1
  Moteur/LConn2 -- Réducteur/LConn1
  Ideal Torque Sensor/RConn1 -- Frottements/LConn1 -- rotor/RConn1 -- Capteur angulaire/LConn1
  PS-Simulink Converter/LConn1 -- Capteur angulaire/RConn3
  PS-Simulink Converter1/LConn1 -- Capteur angulaire/RConn2
  Capteur angulaire/RConn1 -- Frottements/RConn1 -- Moteur/RConn2 -- stator/RConn1

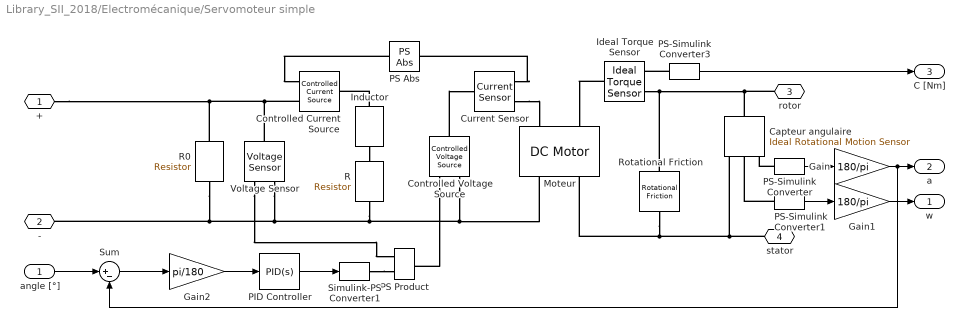
== system Library_SII_2018/Electromécanique/Servomoteur simple ==
  angle [°] : Inport
  Capteur angulaire : fl_lib/Mechanical/Mechanical Sensors/Ideal Rotational Motion Sensor  offset=0 rad
  Controlled Current Source : fl_lib/Electrical/Electrical Sources/Controlled Current Source
  Controlled Voltage Source : fl_lib/Electrical/Electrical Sources/Controlled Voltage Source
  Current Sensor : fl_lib/Electrical/Electrical Sensors/Current Sensor
  Gain : Gain  Gain=180/pi
  Gain1 : Gain  Gain=180/pi
  Gain2 : Gain  Gain=pi/180
  Ideal Torque Sensor : fl_lib/Mechanical/Mechanical Sensors/Ideal Torque Sensor
  Inductor : fl_lib/Electrical/Electrical Elements/Inductor  l=L H  r=0 Ohm  g=1e-9 1/Ohm  i_specify=off  i_priority=High  i=0 A  i_nominal_specify=off  i_nominal_unit=A  i_nominal_value=1  v_specify=off  v_priority=High  v=0 V  v_nominal_specify=off  v_nominal_unit=V  v_nominal_value=1  i_L_specify=off  i_L_priority=High  i_L=0 A  i_L_nominal_specify=off  i_L_nominal_unit=A  i_L_nominal_value=1
  Moteur : elec_lib/Actuators & Drivers/Rotational Actuators/DC Motor  parameterization=1  Ra=R Ohm  La=L H  emf_or_torque=1  Kv=K V/(rad/s)  Ki=6.876e-4 N*m/A  T_stall=2.4e-4 N*m  w_max=1.91e+4 rpm  w_rated=1.5e+4 rpm  P_rated=0.08 W  V_rated=1.5 V  J=0.001 g*cm^2  lam_param=1  lam=kv N*m/(rad/s)  i_noload=0 A  V_i_noload=1.5 V  speed0=0 rpm  alpha=0.00393 1/K  Tmeas=25 C  thermal_mass=100 J/K  initial_temperature=25 C
  PID Controller : simulink/Continuous/PID Controller  Controller=PID  Form=Ideal  TimeDomain=Continuous-time  SampleTime=-1  IntegratorMethod=Forward Euler  FilterMethod=Forward Euler  ControllerParametersSource=internal  P=P  I=I  D=D  UseFilter=on  N=100  TunerSelectOption=Transfer Function Based (PID Tuner App)  InitialConditionSource=internal  InitialConditionForIntegrator=0  InitialConditionForFilter=0  DifferentiatorICPrevScaledInput=0  ExternalReset=none  TrackingMode=off  Kt=1  LimitOutput=on  UpperSaturationLimit=1  LowerSaturationLimit=-1  LinearizeAsGain=on  AntiWindupMode=none  Kb=1  POutMin=[]  POutMax=[]  IOutMin=[]  IOutMax=[]  DOutMin=[]  DOutMax=[]  NOutMin=[]  NOutMax=[]  SumOutMin=[]  SumOutMax=[]  SaturationOutMin=[]  SaturationOutMax=[]  PParamMin=[]  PParamMax=[]  IParamMin=[]  IParamMax=[]  DParamMin=[]  DParamMax=[]  NParamMin=[]  NParamMax=[]  KbParamMin=[]  KbParamMax=[]  KtParamMin=[]  KtParamMax=[]  KbOutMin=[]  KbOutMax=[]  KtOutMin=[]  KtOutMax=[]  IntegratorOutMin=[]  IntegratorOutMax=[]  FilterOutMin=[]  FilterOutMax=[]  SumI1OutMin=[]  SumI1OutMax=[]  SumI2OutMin=[]  SumI2OutMax=[]  SumI3OutMin=[]  SumI3OutMax=[]  SumI4OutMin=[]  SumI4OutMax=[]  SumDOutMin=[]  SumDOutMax=[]  DifferentiatorOutMin=[]  DifferentiatorOutMax=[]  FilterDiffOutCoefMin=[]  FilterDiffOutCoefMax=[]  ReciprocalOutMin=[]  ReciprocalOutMax=[]  SumDenOutMin=[]  SumDenOutMax=[]  SumNumOutMin=[]  SumNumOutMax=[]  DivideOutMin=[]  DivideOutMax=[]  IntegratorContinuousStateAttributes=''  IntegratorStateMustResolveToSignalObject=off  IntegratorRTWStateStorageClass=Auto  FilterContinuousStateAttributes=''  FilterStateMustResolveToSignalObject=off  FilterRTWStateStorageClass=Auto  ParallelPVariant=Passthrough  IdealPVariant=InternalParameters  IVariant=InternalParameters  DVariant=InternalParameters  IntegratorVariant=Continuous  SatVariant=Enabled  AWVariant=Passthrough  PCopyVariant=Disabled  TRVariant=Disabled  FdbkBlocksVariant=Forward  IdealPFdbkVariant=Disabled  SatFdbkVariant=Disabled  DerivativeFilterVariant=ContFilter  NVariant=InternalParameters  NCopyVariant=Disabled  FilterICVariant=InternalICsFilter  IntegratorICVariant=InternalICs  ExternalResetVariant=Disabled  TRSumVariant=Passthrough  SumFdbkVariant=Disabled  SumVariant=Sum_PID
  PS Abs : fl_lib/Physical Signals/Nonlinear Operators/PS Abs
      settings: SourceProductName=Simscape  SourceProductBaseCode=SS
  PS Product : fl_lib/Physical Signals/Functions/PS Product
      settings: SourceProductName=Simscape
  PS-Simulink Converter : nesl_utility/PS-Simulink Converter  PhysicalDomain=network_engine_domain  SubClassName=ps_output  LeftPortType=input  RightPortType=output  PseudoPeriodic=off  Frequencies=[]  Unit=1  AffineConversion=off
  PS-Simulink Converter1 : nesl_utility/PS-Simulink Converter  PhysicalDomain=network_engine_domain  SubClassName=ps_output  LeftPortType=input  RightPortType=output  PseudoPeriodic=off  Frequencies=[]  Unit=1  AffineConversion=off
  PS-Simulink Converter3 : nesl_utility/PS-Simulink Converter  PhysicalDomain=network_engine_domain  SubClassName=ps_output  LeftPortType=input  RightPortType=output  PseudoPeriodic=off  Frequencies=[]  Unit=1  AffineConversion=off
  R : fl_lib/Electrical/Electrical Elements/Resistor  R=R Ohm  i_specify=off  i_priority=High  i=0 A  i_nominal_specify=off  i_nominal_unit=A  i_nominal_value=1  v_specify=off  v_priority=High  v=0 V  v_nominal_specify=off  v_nominal_unit=V  v_nominal_value=1
  R0 : fl_lib/Electrical/Electrical Elements/Resistor  R=R0 Ohm  i_specify=off  i_priority=High  i=0 A  i_nominal_specify=off  i_nominal_unit=A  i_nominal_value=1  v_specify=off  v_priority=High  v=0 V  v_nominal_specify=off  v_nominal_unit=V  v_nominal_value=1
  Rotational Friction : fl_lib/Mechanical/Rotational Elements/Rotational Friction  brkwy_trq=Cf*1.1 N*m  brkwy_vel=0.060623 rad/s  Col_trq=Cf N*m  visc_coef=0.0001 N*m/(rad/s)  w_specify=off  w_priority=High  w=0 rad/s  w_nominal_specify=off  w_nominal_unit=rad/s  w_nominal_value=1  t_specify=off  t_priority=High  t=0 N*m  t_nominal_specify=off  t_nominal_unit=N*m  t_nominal_value=1
      settings: SourceProductName=Simscape
  Simulink-PS Converter1 : nesl_utility/Simulink-PS Converter  PhysicalDomain=network_engine_domain  SubClassName=ps_input  LeftPortType=input  RightPortType=output  PseudoPeriodic=off  Frequencies=[]  NoiseDistribution=none  NoiseParameters=[]  Unit=V  AffineConversion=off  FilteringAndDerivatives=zero  SimscapeFilterOrder=1  InputFilterTimeConstant=0.1  UdotUserProvided=1
  Sum : Sum  Inputs=|+-
  Voltage Sensor : fl_lib/Electrical/Electrical Sensors/Voltage Sensor
  + : PMIOPort  Side=Left
  - : PMIOPort  Port=2  Side=Left
  rotor : PMIOPort  Port=3  Side=Right
  stator : PMIOPort  Port=4  Side=Right
  w : Outport
  a : Outport  Port=2
  C [Nm] : Outport  Port=3
  wires:
  PID Controller/1 -> Simulink-PS Converter1/1
  Gain1/1 -> w/1
  PS-Simulink Converter/1 -> Gain/1
  PS-Simulink Converter1/1 -> Gain1/1
  Gain2/1 -> PID Controller/1
  angle [°]/1 -> Sum/1
  Gain/1 -> Sum/2, a/1
  Sum/1 -> Gain2/1
  PS-Simulink Converter3/1 -> C [Nm]/1
  connections:
  Inductor/RConn1 -- R/LConn1
  Inductor/LConn1 -- Controlled Current Source/LConn1
  Current Sensor/RConn1 -- PS Abs/LConn1
  Current Sensor/RConn2 -- Moteur/LConn1
  Controlled Current Source/RConn2 -- Voltage Sensor/LConn1 -- +/RConn1 -- R0/LConn1
  Controlled Voltage Source/LConn1 -- Current Sensor/LConn1
  Voltage Sensor/RConn2 -- R/RConn1 -- Moteur/RConn1 -- Controlled Voltage Source/RConn2 -- -/RConn1 -- R0/RConn1
  rotor/RConn1 -- Ideal Torque Sensor/RConn1 -- Rotational Friction/LConn1 -- Capteur angulaire/LConn1
  PS-Simulink Converter/LConn1 -- Capteur angulaire/RConn3
  PS-Simulink Converter1/LConn1 -- Capteur angulaire/RConn2
  Capteur angulaire/RConn1 -- Moteur/RConn2 -- Rotational Friction/RConn1 -- stator/RConn1
  Controlled Voltage Source/RConn1 -- PS Product/RConn1
  Simulink-PS Converter1/RConn1 -- PS Product/LConn2
  Voltage Sensor/RConn1 -- PS Product/LConn1
  PS Abs/RConn1 -- Controlled Current Source/RConn1
  Ideal Torque Sensor/LConn1 -- Moteur/LConn2
  PS-Simulink Converter3/LConn1 -- Ideal Torque Sensor/RConn2
